simulink model "DPA_6bitDAC_MIXER_fs32G"  (R2015b)
settings: Solver=FixedStepAuto  SolverMode=SingleTasking  StartTime=0.0  StopTime=1/fs*(4*nn+ni)  FixedStep=1/fs/8  RelTol=1e-3  AbsTol=1e-6
values from neighbouring files (symbols this model uses):
  AM = 1    [load_6bit_DPA_Mixerpsd_fs32G.m]
  DC = 0    [load_6bit_DPA_Mixerpsd_fs32G.m]
  DD = -6    [load_6bit_DPA_Mixerpsd_fs32G.m]
  Fc = 8e9    (= 8000000000)    [load_6bit_DPA_Mixerpsd_fs32G.m]
  fin1 = fs/nn*floor(fin1/fs*nn)    [load_6bit_DPA_Mixerpsd_fs32G.m]
  fin2 = fs/nn*floor(fin2/fs*nn)    [load_6bit_DPA_Mixerpsd_fs32G.m]
  fin3 = fs/nn*floor(fin3/fs*nn)    [load_6bit_DPA_Mixerpsd_fs32G.m]
  fin4 = fs/nn*floor(fin4/fs*nn)    [load_6bit_DPA_Mixerpsd_fs32G.m]
  fin5 = fs/nn*floor(fin5/fs*nn)    [load_6bit_DPA_Mixerpsd_fs32G.m]
  fin6 = fs/nn*floor(fin6/fs*nn)    [load_6bit_DPA_Mixerpsd_fs32G.m]
  fin7 = fs/nn*floor(fin7/fs*nn)    [load_6bit_DPA_Mixerpsd_fs32G.m]
  fin8 = fs/nn*floor(fin8/fs*nn)    [load_6bit_DPA_Mixerpsd_fs32G.m]
  fs = Fc*4    (= 32000000000)    [load_6bit_DPA_Mixerpsd_fs32G.m]
  fsrf = fs*8    (= 256000000000)    [load_6bit_DPA_Mixerpsd_fs32G.m]
settings Model: ExtModeTrigMode=oneshot  ExtModeArmWhenConnect=off  Creator=john  LastModifiedBy=John_dell_NB2019
settings SolverCC: AutoInsertRateTranBlk=on
settings DataIOCC: LimitDataPoints=off  SaveFormat=Array  SignalLoggingSaveFormat=ModelDataLogs
settings OptimizationCC: BlockReduction=off  BooleanDataType=off
settings DebuggingCC: SaveWithParameterizedLinksMsg=none  UnderspecifiedInitializationDetection=Classic  MergeDetectMultiDrivingBlocksExec=none  SignalResolutionControl=TryResolveAllWithWarning  MultiTaskDSMMsg=warning  MultiTaskCondExecSysMsg=none  StateNameClashWarn=warning
settings HardwareCC: ProdBitPerPointer=32  ProdLargestAtomicFloat=None  ProdIntDivRoundTo=Undefined  ProdEndianess=Unspecified  ProdWordSize=32  ProdHWDeviceType=32-bit Generic  TargetBitPerPointer=64  TargetLongLongMode=on  TargetIntDivRoundTo=Zero  TargetEndianess=LittleEndian  TargetWordSize=64  TargetHWDeviceType=MATLAB Host  ProdEqTarget=off
settings GRTTargetCC: GeneratePreprocessorConditionals=Disable all  CombineOutputUpdateFcns=off  GRTInterface=on
settings ConfigComp: CovModelRefEnable=Off

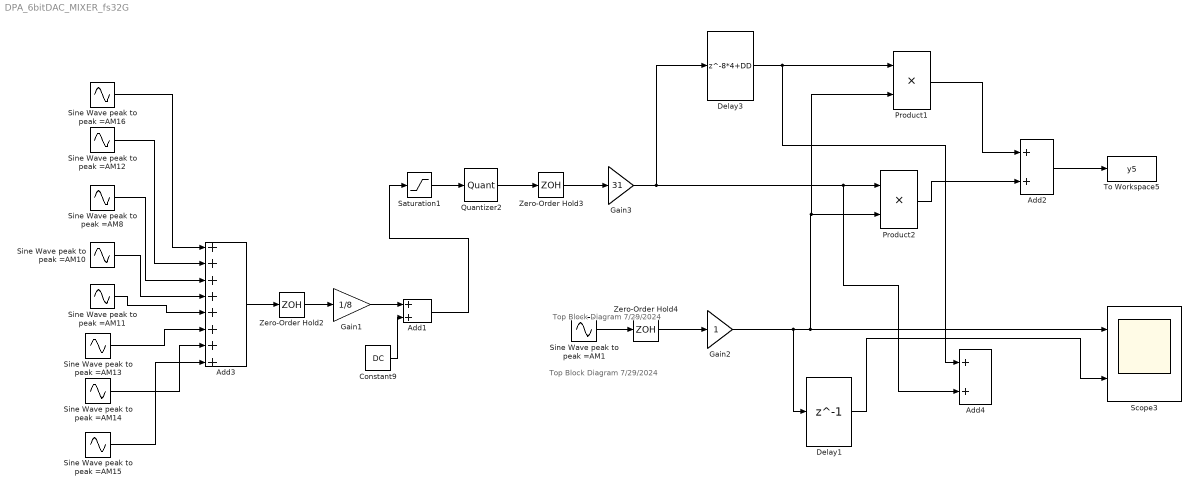
== system DPA_6bitDAC_MIXER_fs32G ==
  note: Top Block Diagram 7/29/2024
  note: Top Block Diagram 7/29/2024
  Add1 : Sum
  Add2 : Sum
  Add3 : Sum  Inputs=++++++++
  Add4 : Sum
  Constant9 : Constant  Value=DC
  Delay1 : Delay  DelayLength=1  InitialCondition=0  SampleTime=1/fs/8
  Delay3 : Delay  DelayLength=8*4+DD  InitialCondition=0  SampleTime=1/fs/8
  Gain1 : Gain  Gain=1/8
  Gain2 : Gain
  Gain3 : Gain  Gain=31
  Product1 : Product
  Product2 : Product
  Quantizer2 : Quantizer  QuantizationInterval=1/2^5  LinearizeAsGain=off
  Saturation1 : Saturate  UpperLimit=1  LowerLimit=-1
  Scope3 : Scope  NumInputPorts=2
  Sine Wave peak to peak =AM1 : Sin  Amplitude=AM  Frequency=2*pi*Fc  Phase=pi/2  SampleTime=2/fs
  Sine Wave peak to peak =AM10 : Sin  Amplitude=AM  Frequency=2*pi*fin4  SampleTime=8/fs
  Sine Wave peak to peak =AM11 : Sin  Amplitude=AM  Frequency=2*pi*fin5  SampleTime=8/fs
  Sine Wave peak to peak =AM12 : Sin  Amplitude=AM  Frequency=2*pi*fin2  SampleTime=8/fs
  Sine Wave peak to peak =AM13 : Sin  Amplitude=AM  Frequency=2*pi*fin6  SampleTime=8/fs
  Sine Wave peak to peak =AM14 : Sin  Amplitude=AM  Frequency=2*pi*fin7  SampleTime=8/fs
  Sine Wave peak to peak =AM15 : Sin  Amplitude=AM  Frequency=2*pi*fin8  SampleTime=8/fs
  Sine Wave peak to peak =AM16 : Sin  Amplitude=AM  Frequency=2*pi*fin1  SampleTime=8/fs
  Sine Wave peak to peak =AM8 : Sin  Amplitude=AM  Frequency=2*pi*fin3  SampleTime=8/fs
  To Workspace5 : ToWorkspace  VariableName=y5  SampleTime=1/fs/8
  Zero-Order Hold2 : ZeroOrderHold  SampleTime=8/fs
  Zero-Order Hold3 : ZeroOrderHold  SampleTime=1/fsrf
  Zero-Order Hold4 : ZeroOrderHold  SampleTime=2/fs
  wires:
  Quantizer2/1 -> Zero-Order Hold3/1
  Zero-Order Hold2/1 -> Gain1/1
  Saturation1/1 -> Quantizer2/1
  Zero-Order Hold3/1 -> Gain3/1
  Gain1/1 -> Add1/1
  Constant9/1 -> Add1/2
  Add1/1 -> Saturation1/1
  Sine Wave peak to peak =AM16/1 -> Add3/1
  Add3/1 -> Zero-Order Hold2/1
  Sine Wave peak to peak =AM12/1 -> Add3/2
  Sine Wave peak to peak =AM8/1 -> Add3/3
  Sine Wave peak to peak =AM10/1 -> Add3/4
  Sine Wave peak to peak =AM11/1 -> Add3/5
  Sine Wave peak to peak =AM13/1 -> Add3/6
  Sine Wave peak to peak =AM14/1 -> Add3/7
  Sine Wave peak to peak =AM15/1 -> Add3/8
  Zero-Order Hold4/1 -> Gain2/1
  Sine Wave peak to peak =AM1/1 -> Zero-Order Hold4/1
  Gain3/1 -> Add4/2, Product2/1, Delay3/1
  Add2/1 -> To Workspace5/1
  Delay1/1 -> Scope3/2
  Gain2/1 -> Delay1/1, Product1/2, Product2/2, Scope3/1
  Product1/1 -> Add2/1
  Product2/1 -> Add2/2
  Delay3/1 -> Add4/1, Product1/1
